simulink model "DriveTrain5MW_DFIG"  (R2019b)
settings: Solver=ode23tb  StartTime=0.0  StopTime=Tend  FixedStep=5e-5  RelTol=1e-3  EnableMultiTasking=on
values from neighbouring files (symbols this model uses):
  D = Lm^2 - Ls*Lr    [DFIG_Control.m]
  DriveTrain5MW = ModalAnalysis(DriveTrain5MW)    [Gearbox5MW_init.m]
  GenModel = SteadyStateDFIG(GenModel)    [DFIG_Control.m]    (also in Gearbox5MW_init.m = MachineDynamicModel(GenModel))
  GridLossTime = 1000    [run_5mw_drivetrain_stand_alone_example.m]
  Id_max = 10.3e4    (= 103000)    [inputGenerator.m]
  Iq_max = 10.3e4    (= 103000)    [inputGenerator.m]
  KQ = 0.01    [inputGenerator.m]
  om_step = 1.1    [run_5mw_drivetrain_stand_alone_example.m]
  omegaWT = 1.88    [Gearbox5MW_init.m]
  po_step = 0    [run_5mw_drivetrain_stand_alone_example.m]
  ss_RefPower = -GenModel.Pn/GenModel.eta    [run_5mw_drivetrain_stand_alone_example.m]
  SwitchFAULT = Tend+1    (= 201)    [run_5mw_drivetrain_stand_alone_example.m]
  SwitchFAULT_Clears = SwitchFAULT + gr.FaultDuration + gr.RecoveryTime    [run_5mw_drivetrain_stand_alone_example.m]
  Tend = 200    [run_5mw_drivetrain_stand_alone_example.m]
  TiQ = 0.1    [inputGenerator.m]
  Ts_sim_F = 1e-3    (= 0.001)    [run_5mw_drivetrain_stand_alone_example.m]
undefined symbols (not defined in the file or in its folder): Tlss0
libraries: simulink x4
Description:
  | This model includes a 3 stage gearbox: one planetary and two parallel. it also includes a dynamic model of a generator.
  | The gearbox model includes the low-speed, intermediate and high-speed shafts stiffness along with the gear mesh stiffness (constant).
settings Model: Creator=jugc  LastModifiedBy=HUSST
settings DataIOCC: SaveFormat=Array  SignalLoggingSaveFormat=ModelDataLogs  SaveOutput=off  SignalLogging=off  ReturnWorkspaceOutputs=off
settings OptimizationCC: ExpressionDepthLimit=2147483647  LifeSpan=inf  SimCompilerOptimization=on
settings DebuggingCC: AlgebraicLoopMsg=error  ArtificialAlgebraicLoopMsg=none  UnderspecifiedInitializationDetection=Classic  MergeDetectMultiDrivingBlocksExec=none  SolverPrmCheckMsg=warning  MultiTaskDSMMsg=warning  MultiTaskCondExecSysMsg=none  FcnCallInpInsideContextMsg=warning  AllowSymbolicDim=off  StateNameClashWarn=warning  SFUnexpectedBacktrackingDiag=warning  SFNoUnconditionalDefaultTransitionDiag=warning  SFExecutionAtInitializationDiag=none  ArithmeticOperatorsInVariantConditions=warning
settings HardwareCC: ProdBitPerPointer=32  ProdBitPerSizeT=32  ProdBitPerPtrDiffT=32  ProdLargestAtomicFloat=None  ProdIntDivRoundTo=Undefined  ProdEndianess=Unspecified  ProdWordSize=32  ProdHWDeviceType=32-bit Generic
settings ModelReferenceCC: PropagateSignalLabelsOutOfModel=off
settings SFSimCC: SFSimEcho=off  SimUseLocalCustomCode=off  CustomCodeUndefinedFunction=UseInterfaceOnly
settings RTWCC: RTWUseLocalCustomCode=off
settings CodeAppCC: StateflowObjectComments=on
settings GRTTargetCC: TargetLangStandard=C89/C90 (ANSI)  GeneratePreprocessorConditionals=Disable all
settings ConfigComp: CovMetricSettings=dw  CovHtmlReporting=on  CovSaveCumulativeToWorkspaceVar=on  CovSaveSingleToWorkspaceVar=on  CovExternalEMLEnable=off  CovSFcnEnable=off
settings ConfigurationSet: Description=SimMechanics 2G

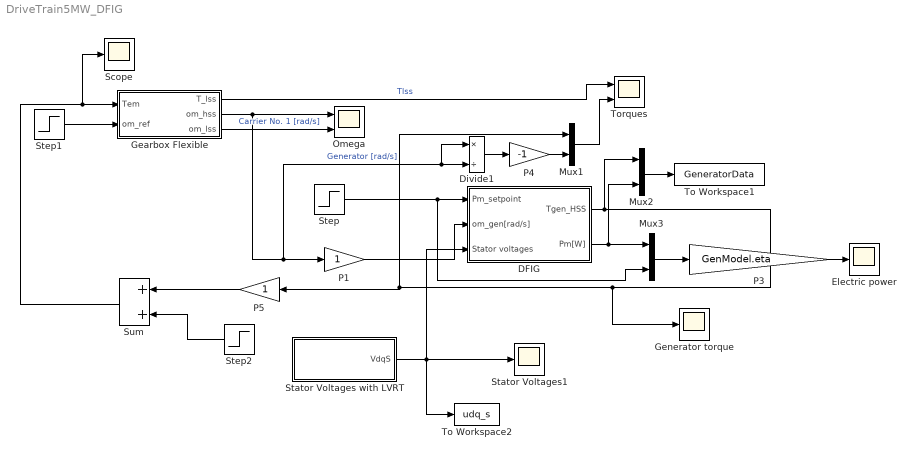
== system DriveTrain5MW_DFIG ==
  DFIG : Subsystem
  Divide1 : Product  Inputs=*/
  Electric power : Scope
  Gearbox Flexible : Subsystem
  Generator torque : Scope
  Mux1 : Mux  Inputs=2
  Mux2 : Mux  Inputs=2
  Mux3 : Mux  Inputs=2
  Omega : Scope  NumInputPorts=2
  P1 : Gain  SaturateOnIntegerOverflow=on  OutDataTypeStr=Inherit: Same as input  ParamDataTypeStr=Inherit: Same as input
  P3 : Gain  Gain=GenModel.eta  SaturateOnIntegerOverflow=on  OutDataTypeStr=Inherit: Same as input  ParamDataTypeStr=Inherit: Same as input
  P4 : Gain  Gain=-1  SaturateOnIntegerOverflow=on  OutDataTypeStr=Inherit: Same as input  ParamDataTypeStr=Inherit: Same as input
  P5 : Gain  SaturateOnIntegerOverflow=on  OutDataTypeStr=Inherit: Same as input  ParamDataTypeStr=Inherit: Same as input
  Scope : Scope
  Stator Voltages with LVRT : Subsystem
  Stator Voltages1 : Scope
  Step : Step  Time=GridLossTime  Before=ss_RefPower  After=po_step  SampleTime=0
  Step1 : Step  Time=40  Before=omegaWT  After=om_step*omegaWT
  Step2 : Step  Time=Tend/2  After=0  SampleTime=0
  Sum : Sum
  To Workspace1 : ToWorkspace  VariableName=GeneratorData  SampleTime=Ts_sim_F
  To Workspace2 : ToWorkspace  VariableName=udq_s  SampleTime=-1
  Torques : Scope  NumInputPorts=2
  wires:
  Step1/1 -> Gearbox Flexible/2("om_ref ")
  Gearbox Flexible/1(T_lss) -> Torques/1  "Tlss"
  Gearbox Flexible/2(om_hss) -> Divide1/1, Divide1/2, P1/1, Omega/1  "Generator [rad/s]"
  Divide1/1 -> P4/1
  Mux2/1 -> To Workspace1/1
  Gearbox Flexible/3(om_lss) -> Omega/2  "Carrier No. 1 [rad/s]"
  P1/1 -> DFIG/2(om_gen[rad/s])
  Mux1/1 -> Torques/2
  DFIG/1(Tgen_HSS) -> Mux2/1, P5/1, Mux1/1, Generator torque/1
  P4/1 -> Mux1/2
  Stator Voltages with LVRT/1(VdqS) -> To Workspace2/1, DFIG/3(Stator voltages), Stator Voltages1/1
  DFIG/2(Pm[W]) -> Mux3/1, Mux2/2
  Mux3/1 -> P3/1
  P3/1 -> Electric power/1
  Step/1 -> Mux3/2, DFIG/1(Pm_setpoint)
  Sum/1 -> Scope/1, Gearbox Flexible/1(Tem)
  P5/1 -> Sum/1
  Step2/1 -> Sum/2

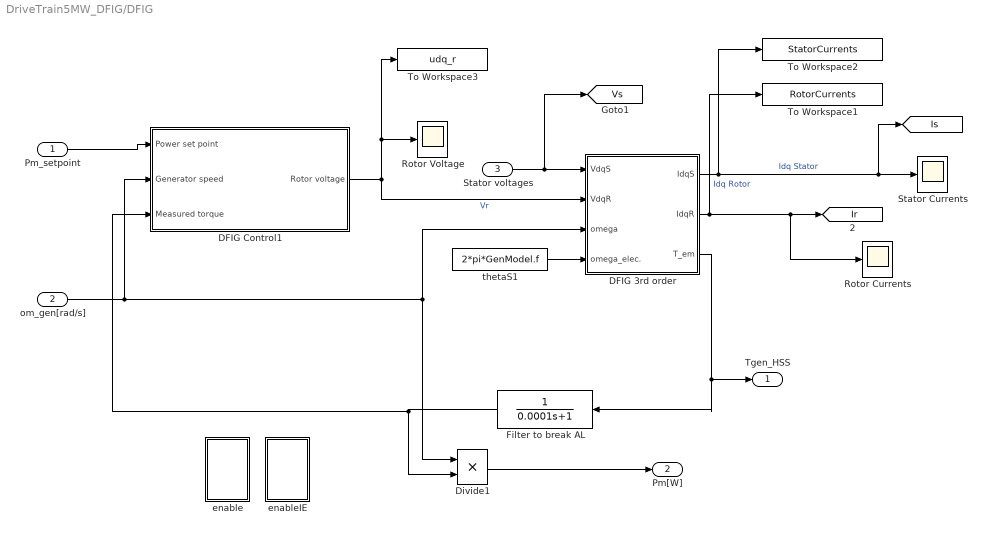
== system DriveTrain5MW_DFIG/DFIG ==
  Pm_setpoint : Inport
  om_gen[rad/s] : Inport  Port=2
  Stator voltages : Inport  Port=3
  DFIG 3rd order : Subsystem
  DFIG Control1 : Subsystem
  Divide1 : Product  Inputs=**
  Filter to break AL : TransferFcn  Denominator=[0.0001 1]
  Rotor Currents : Scope
  "Rotor Voltage " : Scope
  Stator Currents : Scope
  To Workspace1 : ToWorkspace  VariableName=RotorCurrents  SampleTime=-1
  To Workspace2 : ToWorkspace  VariableName=StatorCurrents  SampleTime=-1
  To Workspace3 : ToWorkspace  VariableName=udq_r  SampleTime=-1
  enable : Subsystem
  enableIE : Subsystem
  thetaS1 : Constant  Value=2*pi*GenModel.f
  Tgen_HSS : Outport
  Pm[W] : Outport  Port=2
  tag scope: Ir=global, Is=global, Vs=global
  wires:
  DFIG 3rd order/1(IdqS) -> [Is], Stator Currents/1, To Workspace2/1  "Idq Stator"
  Stator voltages/1 -> DFIG 3rd order/1(VdqS), [Vs]
  Divide1/1 -> Pm[W]/1
  DFIG 3rd order/2(IdqR) -> Rotor Currents/1, [Ir], To Workspace1/1  "Idq Rotor"
  thetaS1/1 -> DFIG 3rd order/4(omega_elec.)
  om_gen[rad/s]/1 -> DFIG Control1/2(Generator speed), DFIG 3rd order/3(omega), Divide1/1
  Pm_setpoint/1 -> DFIG Control1/1(Power set point)
  DFIG Control1/1(Rotor voltage) -> To Workspace3/1, "Rotor Voltage "/1, DFIG 3rd order/2(VdqR)  "Vr"
  DFIG 3rd order/3(T_em) -> Filter to break AL/1, Tgen_HSS/1
  Filter to break AL/1 -> DFIG Control1/3(Measured torque), Divide1/2

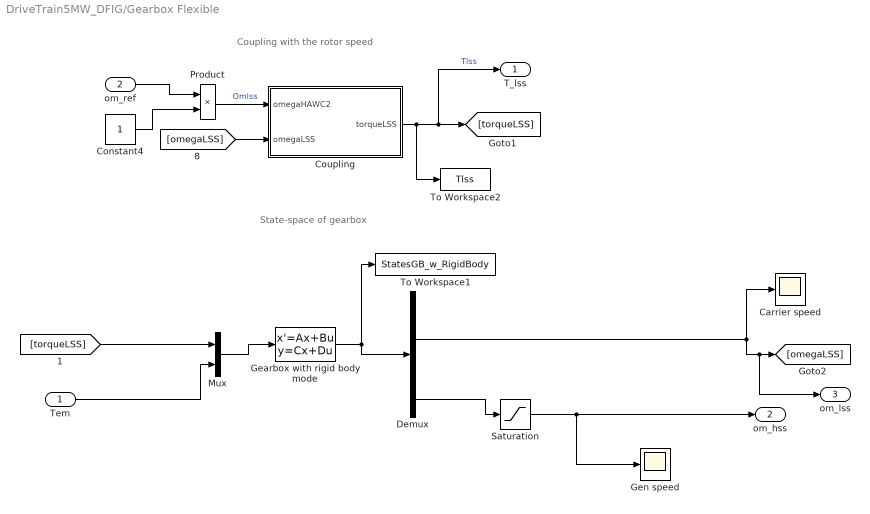
== system DriveTrain5MW_DFIG/Gearbox Flexible ==
  note: Coupling with the rotor speed
  note: State-space of gearbox
  Tem : Inport
  "om_ref " : Inport  Port=2
  Carrier speed : Scope
  Constant4 : Constant
  Coupling : Subsystem
  Demux : Demux  Outputs=DriveTrain5MW.DemuxVec
  Gearbox with rigid body mode : StateSpace  A=DriveTrain5MW.GlobalSys.a  B=DriveTrain5MW.GlobalSys.b  C=DriveTrain5MW.GlobalSys.c  D=DriveTrain5MW.GlobalSys.d  InitialCondition=[DriveTrain5MW.q0Global'; DriveTrain5MW.q0dotGlobal']
  Gen speed : Scope
  Mux : Mux  Inputs=2
  Product : Product
  Saturation : Saturate  UpperLimit=1e3  LowerLimit=-1e3
  To Workspace1 : ToWorkspace  VariableName=StatesGB_w_RigidBody  SampleTime=Ts_sim_F
  To Workspace2 : ToWorkspace  VariableName=Tlss  SampleTime=-1
  T_lss : Outport  InitialOutput=Tlss0
  om_hss : Outport  Port=2
  om_lss : Outport  Port=3
  wires:
  Constant4/1 -> Product/2
  Gearbox with rigid body mode/1 -> Demux/1, To Workspace1/1
  Product/1 -> Coupling/1(omegaHAWC2)  "Omlss"
  "om_ref "/1 -> Product/1
  Tem/1 -> Mux/2
  [omegaLSS] -> Coupling/2(omegaLSS)
  Coupling/1(torqueLSS) -> To Workspace2/1, T_lss/1, [torqueLSS]  "Tlss"
  Demux/2 -> om_lss/1, [omegaLSS], Carrier speed/1
  Demux/4 -> Saturation/1
  Saturation/1 -> om_hss/1, Gen speed/1
  [torqueLSS] -> Mux/1
  Mux/1 -> Gearbox with rigid body mode/1

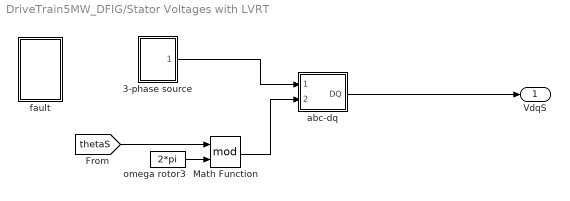
== system DriveTrain5MW_DFIG/Stator Voltages with LVRT ==
  3-phase source : Subsystem  mask(3 - Phase Voltage Source){U=GenModel.Unl, fs=GenModel.f}
      mask prompts: U "Phase voltage Amplitude [V]"; fs "Fundamental frequency [Hz]"
  Math Function : Math  Operator=mod  SaturateOnIntegerOverflow=on
  abc-dq : Subsystem
  fault : Subsystem
  omega rotor3 : Constant  Value=2*pi
  VdqS : Outport
  wires:
  Math Function/1 -> abc-dq/2(theta)
  [thetaS] -> Math Function/1
  omega rotor3/1 -> Math Function/2
  abc-dq/1(DQ) -> VdqS/1
  3-phase source/1(uRST) -> abc-dq/1(ABC)

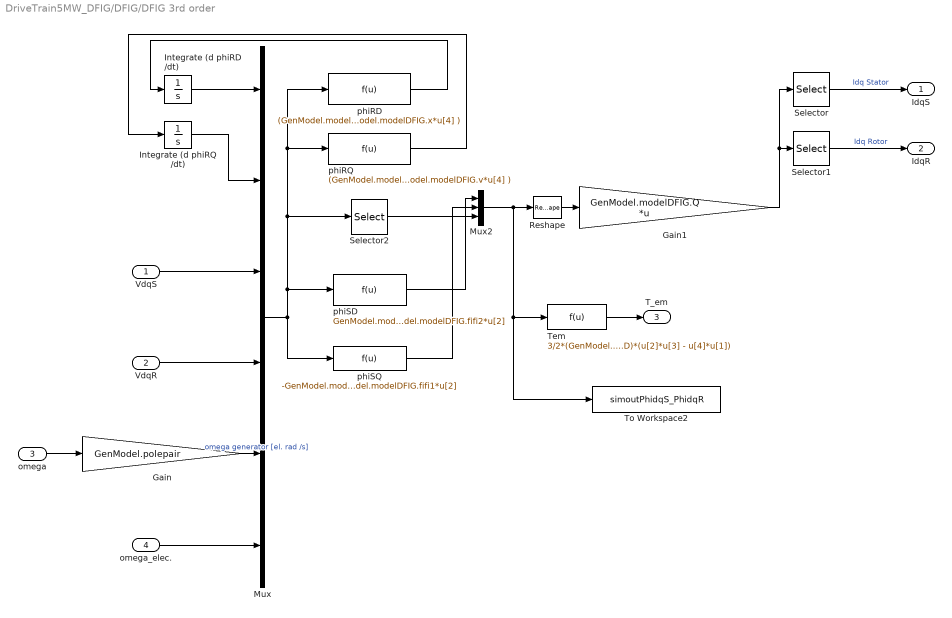
== system DriveTrain5MW_DFIG/DFIG/DFIG 3rd order ==
  VdqS : Inport
  VdqR : Inport  Port=2
  omega : Inport  Port=3
  omega_elec. : Inport  Port=4
  Gain : Gain  Gain=GenModel.polepair
  Gain1 : Gain  Gain=GenModel.modelDFIG.Q  Multiplication=Matrix(K*u)
  Integrate (d phiRD /dt) : Integrator  InitialCondition=GenModel.modelDFIG.x_phi(1)  AbsoluteTolerance=0.01
  Integrate (d phiRQ /dt) : Integrator  InitialCondition=GenModel.modelDFIG.x_phi(2)  AbsoluteTolerance=0.01
  Mux : Mux  Inputs=6
  Mux2 : Mux  Inputs=3
  Reshape : Reshape  OutputDimensionality=Column vector (2-D)
  Selector : Selector  InputPortWidth=4  IndexOptions=Index vector (dialog)  Indices=[1 2]  OutputSizes=1
  Selector1 : Selector  InputPortWidth=4  IndexOptions=Index vector (dialog)  Indices=[3 4]  OutputSizes=1
  Selector2 : Selector  IndexOptions=Index vector (dialog)  Indices=[1 2]  OutputSizes=1
  Tem : Fcn  Expr=3/2*(GenModel.polepair)*(GenModel.modelDFIG.Lm/GenModel.modelDFIG.D)*(u[2]*u[3] - u[4]*u[1])
  To Workspace2 : ToWorkspace  VariableName=simoutPhidqS_PhidqR  SampleTime=-1
  phiRD : Fcn  Expr="(GenModel.modelDFIG.q - GenModel.modelDFIG.RLD)*u[1] + ( GenModel.modelDFIG.w +(u(8) - u[7]) )*u[2]  +  u[5]  - ( GenModel.modelDFIG.z*u[3]  +  GenModel.modelDFIG.x*u[4] )"
  phiRQ : Fcn  Expr="(GenModel.modelDFIG.r - (u[8] - u[7]))*u[1]  +  (GenModel.modelDFIG.t - GenModel.modelDFIG.RLD)*u[2]  +  u[6]  -  ( GenModel.modelDFIG.c*u[3] + GenModel.modelDFIG.v*u[4] )"
  phiSD : Fcn  Expr="GenModel.modelDFIG.fiV1*u[3] + GenModel.modelDFIG.fiV2*u[4]  + GenModel.modelDFIG.fifi1*u[1]  +  GenModel.modelDFIG.fifi2*u[2]"
  phiSQ : Fcn  Expr="-GenModel.modelDFIG.fiV2*u[3] + GenModel.modelDFIG.fiV1*u[4]  - GenModel.modelDFIG.fifi2*u[1]  +  GenModel.modelDFIG.fifi1*u[2]"
  IdqS : Outport
  IdqR : Outport  Port=2
  T_em : Outport  Port=3
  wires:
  omega/1 -> Gain/1
  Tem/1 -> T_em/1
  Selector1/1 -> IdqR/1  "Idq Rotor"
  Selector/1 -> IdqS/1  "Idq Stator"
  Gain1/1 -> Selector1/1, Selector/1
  Reshape/1 -> Gain1/1
  Mux2/1 -> To Workspace2/1, Tem/1, Reshape/1
  Integrate (d phiRQ /dt)/1 -> Mux/2
  Integrate (d phiRD /dt)/1 -> Mux/1
  VdqR/1 -> Mux/4
  VdqS/1 -> Mux/3
  Gain/1 -> Mux/5  "omega generator [el. rad /s]"
  phiRD/1 -> Integrate (d phiRD /dt)/1
  phiRQ/1 -> Integrate (d phiRQ /dt)/1
  Mux/1 -> phiSQ/1, phiSD/1, Selector2/1, phiRD/1, phiRQ/1
  Selector2/1 -> Mux2/3
  phiSD/1 -> Mux2/1
  phiSQ/1 -> Mux2/2
  omega_elec./1 -> Mux/6

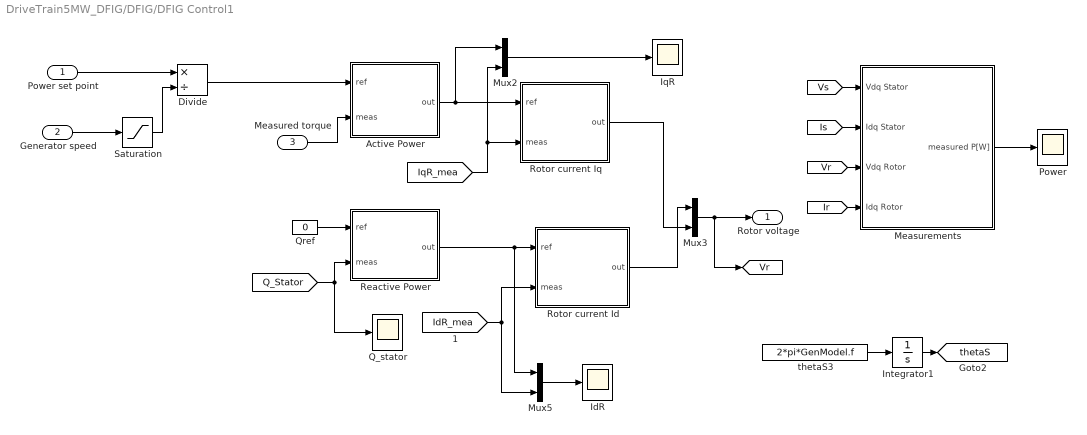
== system DriveTrain5MW_DFIG/DFIG/DFIG Control1 ==
  Power set point : Inport
  Generator speed : Inport  Port=2
  Measured torque : Inport  Port=3
  Active Power : Subsystem
      settings: MinAlgLoopOccurrences=on
  Divide : Product  Inputs=*/
  IdR : Scope
  Integrator1 : Integrator
  IqR : Scope
  Measurements : Subsystem
  Mux2 : Mux  Inputs=2
  Mux3 : Mux  Inputs=2
  Mux5 : Mux  Inputs=2
  Power : Scope
  Q_stator : Scope
  Qref : Constant  Value=0
  Reactive Power : Subsystem
  Rotor current Id : Subsystem
  Rotor current Iq : Subsystem
      settings: MinAlgLoopOccurrences=on
  Saturation : Saturate  UpperLimit=1e4  LowerLimit=0.1
  thetaS3 : Constant  Value=2*pi*GenModel.f  SampleTime=1e-3
  Rotor voltage : Outport
  tag scope: Vr=global, thetaS=global
  wires:
  [Is] -> Measurements/2(Idq Stator)
  [Ir] -> Measurements/4(Idq Rotor)
  [Vs] -> Measurements/1(Vdq Stator)
  [Vr] -> Measurements/3(Vdq Rotor)
  Measurements/1(measured P[W]) -> Power/1
  Measured torque/1 -> Active Power/2(meas)
  Mux3/1 -> Rotor voltage/1, [Vr]
  Rotor current Iq/1(out) -> Mux3/2
  Active Power/1(out) -> Mux2/1, Rotor current Iq/1(ref)
  Rotor current Id/1(out) -> Mux3/1
  [IqR_mea] -> Mux2/2, Rotor current Iq/2(meas)
  Reactive Power/1(out) -> Mux5/1, Rotor current Id/1(ref)
  [Q_Stator] -> Reactive Power/2(meas), Q_stator/1
  Qref/1 -> Reactive Power/1(ref)
  thetaS3/1 -> Integrator1/1
  Integrator1/1 -> [thetaS]
  Mux2/1 -> IqR/1
  [IdR_mea] -> Rotor current Id/2(meas), Mux5/2
  Mux5/1 -> IdR/1
  Power set point/1 -> Divide/1
  Saturation/1 -> Divide/2
  Generator speed/1 -> Saturation/1
  Divide/1 -> Active Power/1(ref)

== system DriveTrain5MW_DFIG/DFIG/enable ==
  " on" : Constant
  Clock : Clock
  Switch : Switch  Threshold=GenModel.controlDFIG.SwitchCTLRon
  off : Constant  Value=0
  tag scope: enable=global
  wires:
  Clock/1 -> Switch/2
  Switch/1 -> [enable]
  off/1 -> Switch/3
  " on"/1 -> Switch/1

== system DriveTrain5MW_DFIG/DFIG/enableIE ==
  " on" : Constant
  Clock : Clock
  Switch : Switch  Threshold=GenModel.controlDFIG.SwitchIE_CTLRon
  off : Constant  Value=0
  tag scope: enableIE=global
  wires:
  Clock/1 -> Switch/2
  Switch/1 -> [enableIE]
  off/1 -> Switch/3
  " on"/1 -> Switch/1

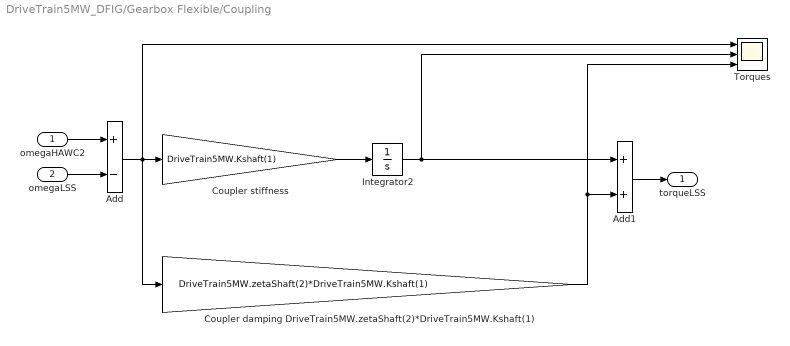
== system DriveTrain5MW_DFIG/Gearbox Flexible/Coupling ==
  omegaHAWC2 : Inport
  omegaLSS : Inport  Port=2
  Add : Sum  Inputs=+-
  Add1 : Sum
  "Coupler damping DriveTrain5MW.zetaShaft(2)*DriveTrain5MW.Kshaft(1) " : Gain  Gain=DriveTrain5MW.zetaShaft(2)*DriveTrain5MW.Kshaft(1)
  Coupler stiffness : Gain  Gain=DriveTrain5MW.Kshaft(1)
  Integrator2 : Integrator  ContinuousStateAttributes='torquelowspeedshaft'
  Torques : Scope  NumInputPorts=3
  torqueLSS : Outport
  wires:
  "Coupler damping DriveTrain5MW.zetaShaft(2)*DriveTrain5MW.Kshaft(1) "/1 -> Add1/2, Torques/3
  Add1/1 -> torqueLSS/1
  Integrator2/1 -> Add1/1, Torques/2
  omegaHAWC2/1 -> Add/1
  omegaLSS/1 -> Add/2
  Add/1 -> Coupler stiffness/1, Torques/1, "Coupler damping DriveTrain5MW.zetaShaft(2)*DriveTrain5MW.Kshaft(1) "/1
  Coupler stiffness/1 -> Integrator2/1

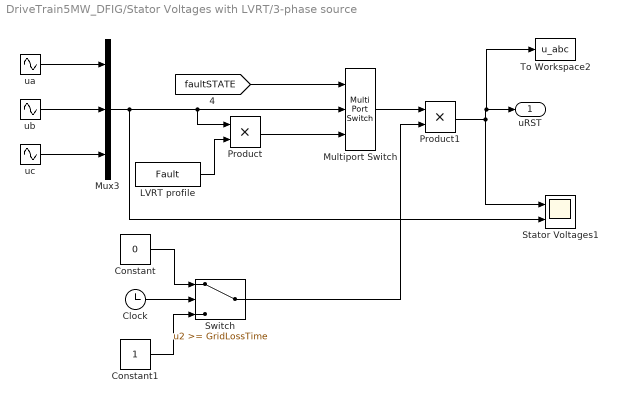
== system DriveTrain5MW_DFIG/Stator Voltages with LVRT/3-phase source ==
  Clock : Clock
  Constant : Constant  Value=0
  Constant1 : Constant
  LVRT profile : FromWorkspace  VariableName=Fault  SampleTime=Ts_sim_F  Interpolate=off  OutputAfterFinalValue=Holding final value
  Multiport Switch : MultiPortSwitch  DataPortOrder=Specify indices  Inputs=2  DataPortIndices={1,0}  DiagnosticForDefault=None
  Mux3 : Mux  Inputs=3
  Product : Product  RndMeth=Zero
  Product1 : Product  RndMeth=Zero
  Stator Voltages1 : Scope  NumInputPorts=2
  Switch : Switch  Threshold=GridLossTime
  To Workspace2 : ToWorkspace  VariableName=u_abc  SampleTime=-1
  ua : Sin  Amplitude=U  Frequency=2*pi*fs
  ub : Sin  Amplitude=U  Frequency=2*pi*fs  Phase=-2*pi/3
  uc : Sin  Amplitude=U  Frequency=2*pi*fs  Phase=2*pi/3
  uRST : Outport  InitialOutput=0
  wires:
  [faultSTATE] -> Multiport Switch/1
  LVRT profile/1 -> Product/2
  Mux3/1 -> Product/1, Multiport Switch/2, Stator Voltages1/2
  ua/1 -> Mux3/1
  ub/1 -> Mux3/2
  uc/1 -> Mux3/3
  Switch/1 -> Product1/2
  Clock/1 -> Switch/2
  Constant/1 -> Switch/1
  Constant1/1 -> Switch/3
  Multiport Switch/1 -> Product1/1
  Product1/1 -> To Workspace2/1, uRST/1, Stator Voltages1/1
  Product/1 -> Multiport Switch/3

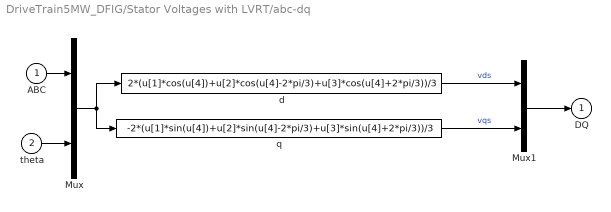
== system DriveTrain5MW_DFIG/Stator Voltages with LVRT/abc-dq ==
  ABC : Inport
  theta : Inport  Port=2
  Mux : Mux  Inputs=[3 1]
  Mux1 : Mux  Inputs=2
  d : Fcn  Expr=2*(u[1]*cos(u[4])+u[2]*cos(u[4]-2*pi/3)+u[3]*cos(u[4]+2*pi/3))/3
  q : Fcn  Expr=-2*(u[1]*sin(u[4])+u[2]*sin(u[4]-2*pi/3)+u[3]*sin(u[4]+2*pi/3))/3
  DQ : Outport  InitialOutput=0
  wires:
  Mux/1 -> d/1, q/1
  ABC/1 -> Mux/1
  d/1 -> Mux1/1  "vds"
  Mux1/1 -> DQ/1
  theta/1 -> Mux/2
  q/1 -> Mux1/2  "vqs"

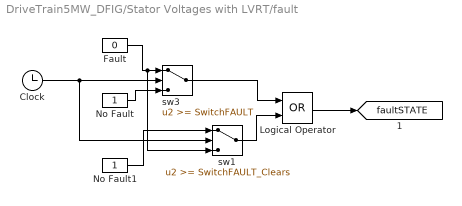
== system DriveTrain5MW_DFIG/Stator Voltages with LVRT/fault ==
  " No Fault" : Constant
  " No Fault1" : Constant
  Clock : Clock
  Fault : Constant  Value=0
  Logical Operator : Logic  Operator=OR  AllPortsSameDT=off  OutDataTypeStr=boolean
  sw1 : Switch  Threshold=SwitchFAULT_Clears
  sw3 : Switch  Threshold=SwitchFAULT
  tag scope: faultSTATE=global
  wires:
  " No Fault1"/1 -> sw1/1
  " No Fault"/1 -> sw3/3
  Fault/1 -> sw3/1, sw1/3
  Logical Operator/1 -> [faultSTATE]
  sw1/1 -> Logical Operator/2
  sw3/1 -> Logical Operator/1
  Clock/1 -> sw3/2, sw1/2

== system DriveTrain5MW_DFIG/DFIG/DFIG Control1/Active Power ==
  ref : Inport
  meas : Inport  Port=2
  Damper3 : simulink/Continuous/PID Controller  Controller=PI  Form=Ideal  TimeDomain=Continuous-time  SampleTime=-1  IntegratorMethod=Forward Euler  FilterMethod=Forward Euler  ControllerParametersSource=internal  P=0.00957890098810026  I=139.222439658911  D=0  UseFilter=on  N=100  TunerSelectOption=Transfer Function Based (PID Tuner App)  InitialConditionSource=internal  InitialConditionForIntegrator=0  InitialConditionForFilter=0  DifferentiatorICPrevScaledInput=0  ExternalReset=none  TrackingMode=off  Kt=1  LimitOutput=off  UpperSaturationLimit=inf  LowerSaturationLimit=-inf  LinearizeAsGain=on  AntiWindupMode=none  Kb=1  POutMin=[]  POutMax=[]  IOutMin=[]  IOutMax=[]  DOutMin=[]  DOutMax=[]  NOutMin=[]  NOutMax=[]  SumOutMin=[]  SumOutMax=[]  SaturationOutMin=[]  SaturationOutMax=[]  PParamMin=[]  PParamMax=[]  IParamMin=[]  IParamMax=[]  DParamMin=[]  DParamMax=[]  NParamMin=[]  NParamMax=[]  KbParamMin=[]  KbParamMax=[]  KtParamMin=[]  KtParamMax=[]  KbOutMin=[]  KbOutMax=[]  KtOutMin=[]  KtOutMax=[]  IntegratorOutMin=[]  IntegratorOutMax=[]  FilterOutMin=[]  FilterOutMax=[]  SumI1OutMin=[]  SumI1OutMax=[]  SumI2OutMin=[]  SumI2OutMax=[]  SumI3OutMin=[]  SumI3OutMax=[]  SumI4OutMin=[]  SumI4OutMax=[]  SumDOutMin=[]  SumDOutMax=[]  DifferentiatorOutMin=[]  DifferentiatorOutMax=[]  FilterDiffOutCoefMin=[]  FilterDiffOutCoefMax=[]  ReciprocalOutMin=[]  ReciprocalOutMax=[]  SumDenOutMin=[]  SumDenOutMax=[]  SumNumOutMin=[]  SumNumOutMax=[]  DivideOutMin=[]  DivideOutMax=[]  IntegratorContinuousStateAttributes=''  IntegratorStateMustResolveToSignalObject=off  IntegratorRTWStateStorageClass=Auto  FilterContinuousStateAttributes=''  FilterStateMustResolveToSignalObject=off  FilterRTWStateStorageClass=Auto  ParallelPVariant=Passthrough  IdealPVariant=InternalParameters  IVariant=InternalParameters  DVariant=Disabled  IntegratorVariant=Continuous  SatVariant=Disabled  AWVariant=Passthrough  PCopyVariant=Disabled  TRVariant=Disabled  FdbkBlocksVariant=Forward  IdealPFdbkVariant=Disabled  SatFdbkVariant=Disabled  DerivativeFilterVariant=Disabled  NVariant=Disabled  NCopyVariant=Disabled_SignalSpec  FilterICVariant=Disabled  IntegratorICVariant=InternalICs  ExternalResetVariant=Disabled  TRSumVariant=Passthrough  SumFdbkVariant=Disabled  SumVariant=Sum_PI
  IdR : Scope
  Sum3 : Sum  Inputs=|+-  SaturateOnIntegerOverflow=on  InputSameDT=on  OutDataTypeStr=Inherit: Same as first input
  out : Outport  InitialOutput=0
  wires:
  Damper3/1 -> out/1, IdR/1
  ref/1 -> Sum3/1
  meas/1 -> Sum3/2
  Sum3/1 -> Damper3/1

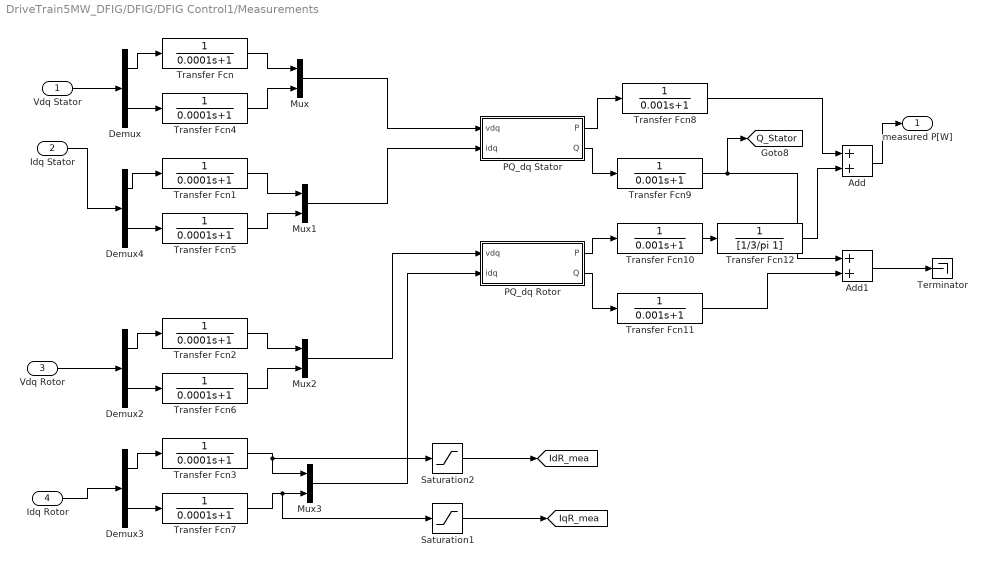
== system DriveTrain5MW_DFIG/DFIG/DFIG Control1/Measurements ==
  Vdq Stator : Inport
  Idq Stator : Inport  Port=2
  Vdq Rotor : Inport  Port=3
  Idq Rotor : Inport  Port=4
  Add : Sum
  Add1 : Sum
  Demux{,2..4} (4 alike) : Demux  Outputs=2
  Mux{,1..3} (4 alike) : Mux  Inputs=2
  PQ_dq Rotor : Subsystem
  PQ_dq Stator : Subsystem
  Saturation1 : Saturate  UpperLimit=Iq_max  LowerLimit=-Iq_max
  Saturation2 : Saturate  UpperLimit=Id_max  LowerLimit=-Id_max
  Terminator : Terminator
  Transfer Fcn{,1..7} (8 alike) : TransferFcn  Denominator=[0.0001 1]
  Transfer Fcn{8..11} (4 alike) : TransferFcn  Denominator=[0.001 1]
  Transfer Fcn12 : TransferFcn  Denominator=[1/3/pi 1]
  measured P[W] : Outport
  tag scope: IdR_mea=global, IqR_mea=global, Q_Stator=global
  wires:
  Saturation2/1 -> [IdR_mea]
  Saturation1/1 -> [IqR_mea]
  Add1/1 -> Terminator/1
  Transfer Fcn3/1 -> Saturation2/1, Mux3/1
  Demux3/1 -> Transfer Fcn3/1
  Transfer Fcn12/1 -> Add/2
  PQ_dq Rotor/1(P) -> Transfer Fcn10/1
  Transfer Fcn10/1 -> Transfer Fcn12/1
  Transfer Fcn11/1 -> Add1/2
  PQ_dq Rotor/2(Q) -> Transfer Fcn11/1
  Transfer Fcn9/1 -> [Q_Stator], Add1/1
  PQ_dq Stator/2(Q) -> Transfer Fcn9/1
  Transfer Fcn8/1 -> Add/1
  Transfer Fcn2/1 -> Mux2/1
  Mux3/1 -> PQ_dq Rotor/2(idq)
  Transfer Fcn6/1 -> Mux2/2
  Mux2/1 -> PQ_dq Rotor/1(vdq)
  Transfer Fcn7/1 -> Mux3/2, Saturation1/1
  Mux/1 -> PQ_dq Stator/1(vdq)
  Mux1/1 -> PQ_dq Stator/2(idq)
  Transfer Fcn5/1 -> Mux1/2
  Transfer Fcn1/1 -> Mux1/1
  Transfer Fcn4/1 -> Mux/2
  Transfer Fcn/1 -> Mux/1
  Idq Rotor/1 -> Demux3/1
  Vdq Rotor/1 -> Demux2/1
  Demux3/2 -> Transfer Fcn7/1
  Demux2/1 -> Transfer Fcn2/1
  Demux2/2 -> Transfer Fcn6/1
  Demux4/1 -> Transfer Fcn1/1
  Demux4/2 -> Transfer Fcn5/1
  Demux/1 -> Transfer Fcn/1
  Demux/2 -> Transfer Fcn4/1
  Idq Stator/1 -> Demux4/1
  Vdq Stator/1 -> Demux/1
  Add/1 -> measured P[W]/1
  PQ_dq Stator/1(P) -> Transfer Fcn8/1

== system DriveTrain5MW_DFIG/DFIG/DFIG Control1/Reactive Power ==
  ref : Inport
  meas : Inport  Port=2
  Damper3 : simulink/Continuous/PID Controller  Controller=PI  Form=Ideal  TimeDomain=Continuous-time  SampleTime=-1  IntegratorMethod=Forward Euler  FilterMethod=Forward Euler  ControllerParametersSource=internal  P=KQ  I=1/TiQ  D=0  UseFilter=on  N=100  TunerSelectOption=Transfer Function Based (PID Tuner App)  InitialConditionSource=internal  InitialConditionForIntegrator=0  InitialConditionForFilter=0  DifferentiatorICPrevScaledInput=0  ExternalReset=none  TrackingMode=off  Kt=1  LimitOutput=off  UpperSaturationLimit=inf  LowerSaturationLimit=-inf  LinearizeAsGain=on  AntiWindupMode=none  Kb=1  POutMin=[]  POutMax=[]  IOutMin=[]  IOutMax=[]  DOutMin=[]  DOutMax=[]  NOutMin=[]  NOutMax=[]  SumOutMin=[]  SumOutMax=[]  SaturationOutMin=[]  SaturationOutMax=[]  PParamMin=[]  PParamMax=[]  IParamMin=[]  IParamMax=[]  DParamMin=[]  DParamMax=[]  NParamMin=[]  NParamMax=[]  KbParamMin=[]  KbParamMax=[]  KtParamMin=[]  KtParamMax=[]  KbOutMin=[]  KbOutMax=[]  KtOutMin=[]  KtOutMax=[]  IntegratorOutMin=[]  IntegratorOutMax=[]  FilterOutMin=[]  FilterOutMax=[]  SumI1OutMin=[]  SumI1OutMax=[]  SumI2OutMin=[]  SumI2OutMax=[]  SumI3OutMin=[]  SumI3OutMax=[]  SumI4OutMin=[]  SumI4OutMax=[]  SumDOutMin=[]  SumDOutMax=[]  DifferentiatorOutMin=[]  DifferentiatorOutMax=[]  FilterDiffOutCoefMin=[]  FilterDiffOutCoefMax=[]  ReciprocalOutMin=[]  ReciprocalOutMax=[]  SumDenOutMin=[]  SumDenOutMax=[]  SumNumOutMin=[]  SumNumOutMax=[]  DivideOutMin=[]  DivideOutMax=[]  IntegratorContinuousStateAttributes=''  IntegratorStateMustResolveToSignalObject=off  IntegratorRTWStateStorageClass=Auto  FilterContinuousStateAttributes=''  FilterStateMustResolveToSignalObject=off  FilterRTWStateStorageClass=Auto  ParallelPVariant=Passthrough  IdealPVariant=InternalParameters  IVariant=InternalParameters  DVariant=Disabled  IntegratorVariant=Continuous  SatVariant=Disabled  AWVariant=Passthrough  PCopyVariant=Disabled  TRVariant=Disabled  FdbkBlocksVariant=Forward  IdealPFdbkVariant=Disabled  SatFdbkVariant=Disabled  DerivativeFilterVariant=Disabled  NVariant=Disabled  NCopyVariant=Disabled_SignalSpec  FilterICVariant=Disabled  IntegratorICVariant=InternalICs  ExternalResetVariant=Disabled  TRSumVariant=Passthrough  SumFdbkVariant=Disabled  SumVariant=Sum_PI
  Sum3 : Sum  Inputs=|+-  SaturateOnIntegerOverflow=on  InputSameDT=on  OutDataTypeStr=Inherit: Same as first input
  out : Outport  InitialOutput=0
  wires:
  Sum3/1 -> Damper3/1
  ref/1 -> Sum3/1
  meas/1 -> Sum3/2
  Damper3/1 -> out/1

== system DriveTrain5MW_DFIG/DFIG/DFIG Control1/Rotor current Id ==
  ref : Inport
  meas : Inport  Port=2
  Damper3 : simulink/Continuous/PID Controller  Controller=PI  Form=Ideal  TimeDomain=Continuous-time  SampleTime=-1  IntegratorMethod=Forward Euler  FilterMethod=Forward Euler  ControllerParametersSource=internal  P=0.0171332427828938  I=10.7511072442759  D=0  UseFilter=on  N=100  TunerSelectOption=Transfer Function Based (PID Tuner App)  InitialConditionSource=internal  InitialConditionForIntegrator=0  InitialConditionForFilter=0  DifferentiatorICPrevScaledInput=0  ExternalReset=none  TrackingMode=off  Kt=1  LimitOutput=off  UpperSaturationLimit=inf  LowerSaturationLimit=-inf  LinearizeAsGain=on  AntiWindupMode=none  Kb=1  POutMin=[]  POutMax=[]  IOutMin=[]  IOutMax=[]  DOutMin=[]  DOutMax=[]  NOutMin=[]  NOutMax=[]  SumOutMin=[]  SumOutMax=[]  SaturationOutMin=[]  SaturationOutMax=[]  PParamMin=[]  PParamMax=[]  IParamMin=[]  IParamMax=[]  DParamMin=[]  DParamMax=[]  NParamMin=[]  NParamMax=[]  KbParamMin=[]  KbParamMax=[]  KtParamMin=[]  KtParamMax=[]  KbOutMin=[]  KbOutMax=[]  KtOutMin=[]  KtOutMax=[]  IntegratorOutMin=[]  IntegratorOutMax=[]  FilterOutMin=[]  FilterOutMax=[]  SumI1OutMin=[]  SumI1OutMax=[]  SumI2OutMin=[]  SumI2OutMax=[]  SumI3OutMin=[]  SumI3OutMax=[]  SumI4OutMin=[]  SumI4OutMax=[]  SumDOutMin=[]  SumDOutMax=[]  DifferentiatorOutMin=[]  DifferentiatorOutMax=[]  FilterDiffOutCoefMin=[]  FilterDiffOutCoefMax=[]  ReciprocalOutMin=[]  ReciprocalOutMax=[]  SumDenOutMin=[]  SumDenOutMax=[]  SumNumOutMin=[]  SumNumOutMax=[]  DivideOutMin=[]  DivideOutMax=[]  IntegratorContinuousStateAttributes=''  IntegratorStateMustResolveToSignalObject=off  IntegratorRTWStateStorageClass=Auto  FilterContinuousStateAttributes=''  FilterStateMustResolveToSignalObject=off  FilterRTWStateStorageClass=Auto  ParallelPVariant=Passthrough  IdealPVariant=InternalParameters  IVariant=InternalParameters  DVariant=Disabled  IntegratorVariant=Continuous  SatVariant=Disabled  AWVariant=Passthrough  PCopyVariant=Disabled  TRVariant=Disabled  FdbkBlocksVariant=Forward  IdealPFdbkVariant=Disabled  SatFdbkVariant=Disabled  DerivativeFilterVariant=Disabled  NVariant=Disabled  NCopyVariant=Disabled_SignalSpec  FilterICVariant=Disabled  IntegratorICVariant=InternalICs  ExternalResetVariant=Disabled  TRSumVariant=Passthrough  SumFdbkVariant=Disabled  SumVariant=Sum_PI
  Sum3 : Sum  Inputs=|+-  SaturateOnIntegerOverflow=on  InputSameDT=on  OutDataTypeStr=Inherit: Same as first input
  out : Outport  InitialOutput=0
  wires:
  ref/1 -> Sum3/1
  meas/1 -> Sum3/2
  Damper3/1 -> out/1
  Sum3/1 -> Damper3/1

== system DriveTrain5MW_DFIG/DFIG/DFIG Control1/Rotor current Iq ==
  ref : Inport
  meas : Inport  Port=2
  Damper3 : simulink/Continuous/PID Controller  Controller=PI  Form=Ideal  TimeDomain=Continuous-time  SampleTime=-1  IntegratorMethod=Forward Euler  FilterMethod=Forward Euler  ControllerParametersSource=internal  P=0.435207128511693  I=202.904901169888  D=0  UseFilter=on  N=100  TunerSelectOption=Transfer Function Based (PID Tuner App)  InitialConditionSource=internal  InitialConditionForIntegrator=0  InitialConditionForFilter=0  DifferentiatorICPrevScaledInput=0  ExternalReset=none  TrackingMode=off  Kt=1  LimitOutput=off  UpperSaturationLimit=inf  LowerSaturationLimit=-inf  LinearizeAsGain=on  AntiWindupMode=none  Kb=1  POutMin=[]  POutMax=[]  IOutMin=[]  IOutMax=[]  DOutMin=[]  DOutMax=[]  NOutMin=[]  NOutMax=[]  SumOutMin=[]  SumOutMax=[]  SaturationOutMin=[]  SaturationOutMax=[]  PParamMin=[]  PParamMax=[]  IParamMin=[]  IParamMax=[]  DParamMin=[]  DParamMax=[]  NParamMin=[]  NParamMax=[]  KbParamMin=[]  KbParamMax=[]  KtParamMin=[]  KtParamMax=[]  KbOutMin=[]  KbOutMax=[]  KtOutMin=[]  KtOutMax=[]  IntegratorOutMin=[]  IntegratorOutMax=[]  FilterOutMin=[]  FilterOutMax=[]  SumI1OutMin=[]  SumI1OutMax=[]  SumI2OutMin=[]  SumI2OutMax=[]  SumI3OutMin=[]  SumI3OutMax=[]  SumI4OutMin=[]  SumI4OutMax=[]  SumDOutMin=[]  SumDOutMax=[]  DifferentiatorOutMin=[]  DifferentiatorOutMax=[]  FilterDiffOutCoefMin=[]  FilterDiffOutCoefMax=[]  ReciprocalOutMin=[]  ReciprocalOutMax=[]  SumDenOutMin=[]  SumDenOutMax=[]  SumNumOutMin=[]  SumNumOutMax=[]  DivideOutMin=[]  DivideOutMax=[]  IntegratorContinuousStateAttributes=''  IntegratorStateMustResolveToSignalObject=off  IntegratorRTWStateStorageClass=Auto  FilterContinuousStateAttributes=''  FilterStateMustResolveToSignalObject=off  FilterRTWStateStorageClass=Auto  ParallelPVariant=Passthrough  IdealPVariant=InternalParameters  IVariant=InternalParameters  DVariant=Disabled  IntegratorVariant=Continuous  SatVariant=Disabled  AWVariant=Passthrough  PCopyVariant=Disabled  TRVariant=Disabled  FdbkBlocksVariant=Forward  IdealPFdbkVariant=Disabled  SatFdbkVariant=Disabled  DerivativeFilterVariant=Disabled  NVariant=Disabled  NCopyVariant=Disabled_SignalSpec  FilterICVariant=Disabled  IntegratorICVariant=InternalICs  ExternalResetVariant=Disabled  TRSumVariant=Passthrough  SumFdbkVariant=Disabled  SumVariant=Sum_PI
  Sum3 : Sum  Inputs=|+-  SaturateOnIntegerOverflow=on  InputSameDT=on  OutDataTypeStr=Inherit: Same as first input
  out : Outport  InitialOutput=0
  wires:
  Sum3/1 -> Damper3/1
  ref/1 -> Sum3/1
  meas/1 -> Sum3/2
  Damper3/1 -> out/1

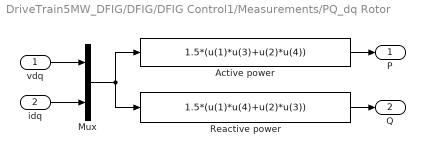
== system DriveTrain5MW_DFIG/DFIG/DFIG Control1/Measurements/PQ_dq Rotor ==
  vdq : Inport
  idq : Inport  Port=2
  Active power : Fcn  Expr=1.5*(u(1)*u(3)+u(2)*u(4))
  Mux : Mux  Inputs=[2 2]
  Reactive power : Fcn  Expr=1.5*(u(1)*u(4)+u(2)*u(3))
  P : Outport
  Q : Outport  Port=2
  wires:
  Mux/1 -> Active power/1, Reactive power/1
  vdq/1 -> Mux/1
  idq/1 -> Mux/2
  Active power/1 -> P/1
  Reactive power/1 -> Q/1

== system DriveTrain5MW_DFIG/DFIG/DFIG Control1/Measurements/PQ_dq Stator ==
  vdq : Inport
  idq : Inport  Port=2
  Active power : Fcn  Expr=1.5*(u(1)*u(3)+u(2)*u(4))
  Mux : Mux  Inputs=[2 2]
  Reactive power : Fcn  Expr=1.5*(u(1)*u(4)+u(2)*u(3))
  P : Outport
  Q : Outport  Port=2
  wires:
  Mux/1 -> Active power/1, Reactive power/1
  vdq/1 -> Mux/1
  idq/1 -> Mux/2
  Active power/1 -> P/1
  Reactive power/1 -> Q/1
